simulink model "envelope_detection_hilbert_with_filter_designer_v5"  (R2021b)
settings: Solver=VariableStepAuto  StartTime=0.0  StopTime=5  FixedStep=5e-07  RelTol=1e-3
libraries: dsparch4 x2, dspvision x2, commanapbnd3 x1, commchan3 x1, spsMeanLib x1
settings Model: Creator=caccolillo  LastModifiedBy=caccolillo

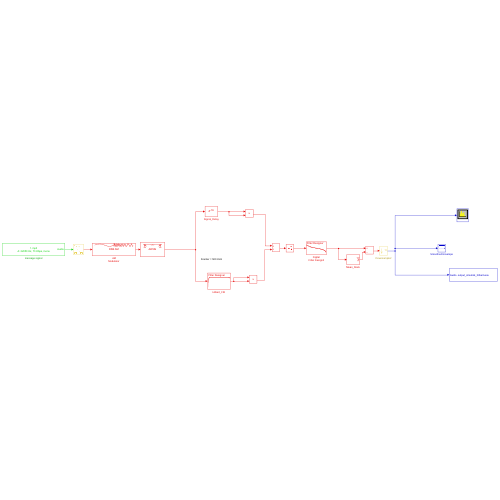
[thumbnail: Simulink's stored preview of the top-level diagram]
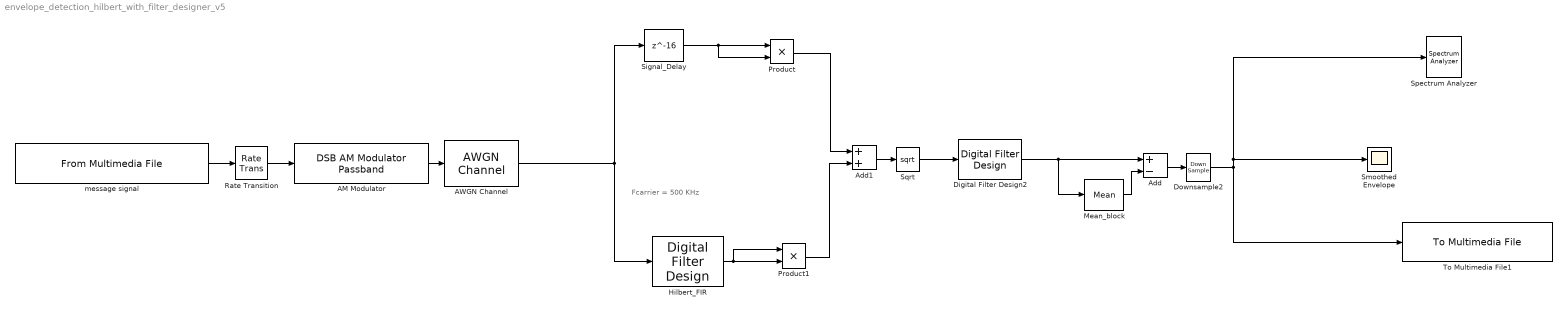
== system envelope_detection_hilbert_with_filter_designer_v5 ==
  note: Fcarrier = 500 KHz
  " AM Modulator " : commanapbnd3/DSB AM Modulator Passband  Fc=500000  Ph=0  Offset=1
      settings: SourceProductBaseCode=CM
  AWGN Channel : commchan3/AWGN Channel  InputProcessing=Columns as channels (frame based)  seed=67  noiseMode="Signal to noise ratio  (Eb/No)"  EbNodB=75  EsNodB=10  SNRdB=10  bitsPerSym=1  Ps=1  Tsym=1  variance=1
  Add : Sum  Inputs=+-
  Add1 : Sum
  Digital Filter Design2 : dsparch4/Digital Filter Design  mwdsp_browser_bugfix_var=off
  Downsample2 : DownSample  N=15  RateOptions=Allow multirate processing
  Hilbert_FIR : dsparch4/Digital Filter Design  mwdsp_browser_bugfix_var=off
  Mean_block : spsMeanLib/Mean  Freq=60  Vinit=0  Ts=1e-05
  Product : Product
  Product1 : Product
  Rate Transition : RateTransition  Deterministic=off
  Signal_Delay : Delay  DelayLength=16
  Smoothed Envelope : Scope
  Spectrum Analyzer : SpectrumAnalyzer
  Sqrt : Sqrt  SaturateOnIntegerOverflow=on
  To Multimedia File1 : dspvision/To Multimedia File  outputFilename=./output_simulink_hilbert.wav  streamSelection=Audio only  videoCompressor=None (uncompressed)  audioCompressor=None (uncompressed)  imagePorts=Separate color signals  fileType=WAV  audioDatatype=16-bit integer  fourcc=RGB  videoQuality=75  mj2000CompFactor=10
  message signal : dspvision/From Multimedia File  inputFilename=/home/caccolillo/hilbert_transform_am/audio/1.mp3  readRange=[1 Inf]  loop=on  numPlays=inf  outputStreams=Audio only  videoDataType=single  audioDataType=double  inheritSampleTime=on  userDefinedSampleTime=5.0E-7  noAudioOutput=off  isIntensityVideo=off  fourcc=RGB  colorVideoFormat=Separate color signals  outputEOF=off  dataOrg=Column-major  audioFrameSize=1  computeAudioFrameSize=off  outSamplingMode=Frame based
  wires:
  AWGN Channel/1 -> Signal_Delay/1, Hilbert_FIR/1
  Add/1 -> Downsample2/1
  Sqrt/1 -> Digital Filter Design2/1
  Hilbert_FIR/1 -> Product1/2, Product1/1
  Signal_Delay/1 -> Product/1, Product/2
  message signal/1 -> Rate Transition/1
  Rate Transition/1 -> " AM Modulator "/1
  " AM Modulator "/1 -> AWGN Channel/1
  Mean_block/1 -> Add/2
  Add1/1 -> Sqrt/1
  Product/1 -> Add1/1
  Product1/1 -> Add1/2
  Digital Filter Design2/1 -> Add/1, Mean_block/1
  Downsample2/1 -> Smoothed Envelope/1, Spectrum Analyzer/1, To Multimedia File1/1
